simulink model "Joint_Control_r2007a"  (Simulink 6.0)
settings: Solver=ode1  StartTime=0.0  StopTime=inf  FixedStep=0.001  RelTol=1e-3
undefined symbols (not defined in the file): HIL, qc_get_step_size
libraries: simulink x6, quarc_library x3
settings Model: Creator=RSamra  LastModifiedBy=ajavid  SimulationMode=external  ExtModeTrigDuration=10000
settings SolverCC: PositivePriorityOrder=on
settings OptimizationCC: InlineInvariantSignals=off  ExpressionDepthLimit=2147483647  SimCompilerOptimization=Off
settings DebuggingCC: SignalResolutionControl=UseLocalSettings  FcnCallInpInsideContextMsg=Use local settings  StateNameClashWarn=warning  StrictBusMsg=Warning
settings HardwareCC: TargetHWDeviceType=32-bit Generic
settings RTWCC: SystemTargetFile=quarc_windows.tlc  TemplateMakefile=quarc_default_tmf  Description=QuaRC Win32 Target  ProcessScript=quarc_windows_make_rtw_hook  RTWCompilerOptimization=Off
settings CodeAppCC: CustomSymbolStrType=$N$R$M
settings STFCustomTargetCC: TargetFcnLib=ansi_tfl_tmw.mat  TargetPreCompLibLocation=C:\DOCUME~1\ALLUSE~1\APPLIC~1\QuaRC\lib\2007b\windows\release  GenFloatMathFcnCalls=ANSI_C  SystemTargetFile=quarc_windows.tlc
settings GRTTargetCC: TargetPreCompLibLocation=C:\DOCUME~1\ALLUSE~1\APPLIC~1\QuaRC\lib\2007b\windows\release  CompOptLevelCompliant=off  MatFileLogging=off  ExtMode=on  ExtModeMexFile=quarc_comm

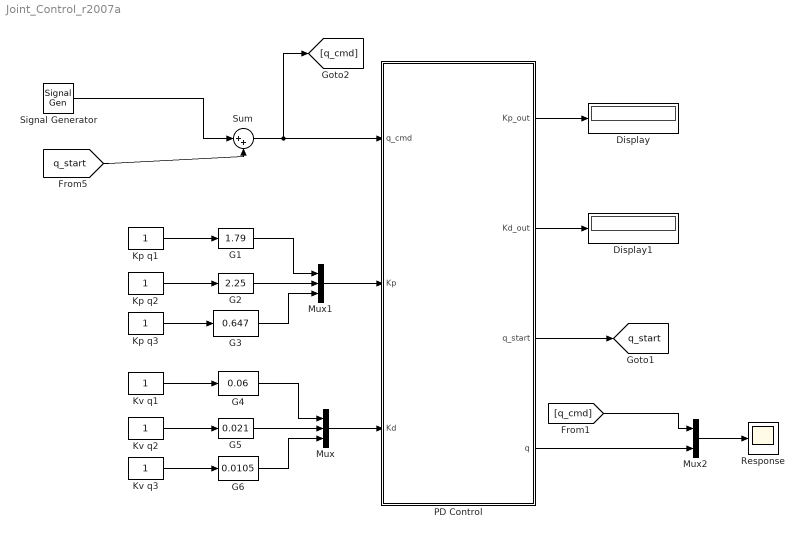
== system Joint_Control_r2007a ==
  Display : Display
  Display1 : Display
  G1 : simulink/Math Operations/Slider Gain  SystemSampleTime=-1  low=0  gain=1.79  high=2
  G2 : simulink/Math Operations/Slider Gain  SystemSampleTime=-1  low=0  gain=2.25  high=3
  G3 : simulink/Math Operations/Slider Gain  SystemSampleTime=-1  low=0  gain=0.647  high=1
  G4 : simulink/Math Operations/Slider Gain  SystemSampleTime=-1  low=0.02  gain=0.06  high=0.1
  G5 : simulink/Math Operations/Slider Gain  SystemSampleTime=-1  low=0.02  gain=0.021  high=0.1
  G6 : simulink/Math Operations/Slider Gain  SystemSampleTime=-1  low=0  gain=0.0105  high=0.025
  Kp q1 : Constant  OutDataType=sfix(16)  OutScaling=2^0
  Kp q2 : Constant  OutDataType=sfix(16)  OutScaling=2^0
  Kp q3 : Constant  OutDataType=sfix(16)  OutScaling=2^0
  Kv q1 : Constant  OutDataType=sfix(16)  OutScaling=2^0
  Kv q2 : Constant  OutDataType=sfix(16)  OutScaling=2^0
  Kv q3 : Constant  OutDataType=sfix(16)  OutScaling=2^0
  Mux : Mux  Inputs=3
  Mux1 : Mux  Inputs=3
  Mux2 : Mux  Inputs=2
  PD Control : Subsystem
  Response : Scope
      settings: TimeRange=50  YMin=-1.25  YMax=3.75
  Signal Generator : SignalGenerator  WaveForm=square  Amplitude=[pi/18 0 0]  Frequency=0.5
  Sum : Sum  Inputs=|++  OutDataType=sfix(16)  OutScaling=2^0
  tag scope: q_start=global
  wires:
  PD Control/3(q_start) -> [q_start]
  Mux2/1 -> Response/1
  Sum/1 -> [q_cmd], PD Control/1(q_cmd)
  [q_start] -> Sum/2
  Signal Generator/1 -> Sum/1
  [q_cmd] -> Mux2/1
  PD Control/4(q) -> Mux2/2
  PD Control/1(Kp_out) -> Display/1
  PD Control/2(Kd_out) -> Display1/1
  Mux/1 -> PD Control/3(Kd)
  Mux1/1 -> PD Control/2(Kp)
  Kp q1/1 -> G1/1
  Kp q2/1 -> G2/1
  Kp q3/1 -> G3/1
  Kv q1/1 -> G4/1
  Kv q2/1 -> G5/1
  Kv q3/1 -> G6/1
  G1/1 -> Mux1/1
  G2/1 -> Mux1/2
  G3/1 -> Mux1/3
  G4/1 -> Mux/1
  G5/1 -> Mux/2
  G6/1 -> Mux/3

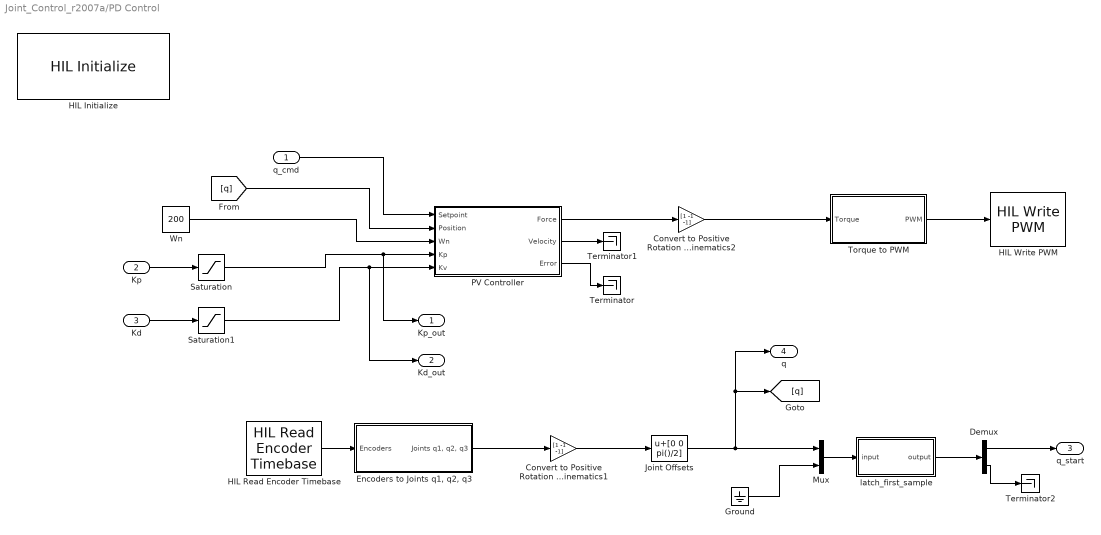
== system Joint_Control_r2007a/PD Control ==
  q_cmd : Inport  OutDataType=sfix(16)  OutScaling=2^0
  Kp : Inport  Port=2  OutDataType=sfix(16)  OutScaling=2^0
  Kd : Inport  Port=3  OutDataType=sfix(16)  OutScaling=2^0
  Convert to Positive Rotation Convension Used in Kinematics1 : Gain  Gain=[1 -1 -1]  ParameterDataType=sfix(16)  ParameterScaling=2^0  OutDataType=sfix(16)  OutScaling=2^0
  Convert to Positive Rotation Convension Used in Kinematics2 : Gain  Gain=[1 -1 -1]  ParameterDataType=sfix(16)  ParameterScaling=2^0  OutDataType=sfix(16)  OutScaling=2^0
  Demux : Demux  Outputs=2
  "Encoders to Joints q1, q2, q3" : Subsystem
  Ground : Ground
  HIL Initialize : quarc_library/Data Acquisition/Generic/Configuration/HIL Initialize  object_name=HIL-3  board_type=phantom_omni  board_number=0  active=on  hardware_clocks=[]  clock_modes=[]  set_clock_params_at_start=off  set_clock_params_at_switch_in=off  analog_input_channels=0:1  analog_input_maximums=10  analog_input_minimums=-10  set_analog_input_params_at_start=off  set_analog_input_params_at_switch_in=off  analog_output_channels=[]  analog_output_maximums=[]  analog_output_minimums=[]  initial_analog_outputs=[]  final_analog_outputs=[]  watchdog_analog_outputs=0  set_analog_output_params_at_start=off  set_analog_output_params_at_switch_in=off  set_analog_outputs_at_start=off  set_analog_outputs_at_switch_in=off  set_analog_outputs_at_terminate=off  set_analog_outputs_at_switch_out=off  set_analog_outputs_on_watchdog=off  digital_input_channels=[]  digital_output_channels=[]  initial_digital_outputs=[]  final_digital_outputs=[]  watchdog_digital_outputs=0  set_digital_outputs_at_start=off  set_digital_outputs_at_switch_in=off  set_digital_outputs_at_terminate=off  set_digital_outputs_at_switch_out=off  set_digital_outputs_on_watchdog=off  encoder_channels=0:2  quadrature=[]  encoder_filter_frequency=[]  initial_encoder_counts=0  set_encoder_params_at_start=off  set_encoder_params_at_switch_in=off  set_encoder_counts_at_start=off  set_encoder_counts_at_switch_in=off  pwm_channels=0:2  pwm_modes=[]  pwm_frequency=[]  initial_pwm_outputs=0  final_pwm_outputs=0  watchdog_pwm_outputs=0  set_pwm_params_at_start=off  set_pwm_params_at_switch_in=off  set_pwm_outputs_at_start=on  set_pwm_outputs_at_switch_in=off  set_pwm_outputs_at_terminate=on  set_pwm_outputs_at_switch_out=off  set_pwm_outputs_on_watchdog=off  other_output_channels=[]  initial_other_outputs=[]  final_other_outputs=[]  watchdog_other_outputs=0  set_other_outputs_at_start=off  set_other_outputs_at_switch_in=off  set_other_outputs_at_terminate=off  set_other_outputs_at_switch_out=off  set_other_outputs_on_watchdog=off
  HIL Read Encoder Timebase : quarc_library/Data Acquisition/Generic/Timebases/HIL Read Encoder Timebase  object_name=HIL-3  clock=0  channels=0:2  samples_in_buffer=max(ceil(1/qc_get_step_size), 1)  active=on  vector_output=on  data_type_mode=Inherit via back propagation  data_type=double
  HIL Write PWM : quarc_library/Data Acquisition/Generic/Immediate I//O/HIL Write PWM  object_name=HIL-3  channels=0:2  sample_time=-1  active=off  vector_input=on
      settings: AttributesFormatString=(%<object_name>)
  Joint Offsets : Bias  Bias=[0 0 pi()/2]
  Mux : Mux  Inputs=2
  PV Controller : Subsystem
  Saturation : Saturate  UpperLimit=[2 2 1]  LowerLimit=[0 0 0]
  Saturation1 : Saturate  UpperLimit=[.1 .1 .025]  LowerLimit=[.02 .02 0]
  Terminator : Terminator
  Terminator1 : Terminator
  Terminator2 : Terminator
  Torque to PWM : Subsystem
  Wn : Constant  Value=200  OutDataType=sfix(16)  OutScaling=2^0
  latch_first_sample : Subsystem
  Kp_out : Outport  OutDataType=sfix(16)  OutScaling=2^0
  Kd_out : Outport  Port=2  OutDataType=sfix(16)  OutScaling=2^0
  q_start : Outport  Port=3  OutDataType=sfix(16)  OutScaling=2^0
  q : Outport  Port=4  OutDataType=sfix(16)  OutScaling=2^0
  wires:
  [q] -> PV Controller/2(Position)
  Wn/1 -> PV Controller/3(Wn)
  Demux/1 -> q_start/1
  Mux/1 -> latch_first_sample/1(input)
  latch_first_sample/1(output) -> Demux/1
  PV Controller/1(Force) -> Convert to Positive Rotation Convension Used in Kinematics2/1
  PV Controller/3(Error) -> Terminator/1
  PV Controller/2(Velocity) -> Terminator1/1
  Ground/1 -> Mux/2
  Demux/2 -> Terminator2/1
  q_cmd/1 -> PV Controller/1(Setpoint)
  Convert to Positive Rotation Convension Used in Kinematics2/1 -> Torque to PWM/1(Torque)
  Convert to Positive Rotation Convension Used in Kinematics1/1 -> Joint Offsets/1
  Joint Offsets/1 -> Mux/1, [q], q/1
  Torque to PWM/1(PWM) -> HIL Write PWM/1
  HIL Read Encoder Timebase/1 -> "Encoders to Joints q1, q2, q3"/1(Encoders)
  "Encoders to Joints q1, q2, q3"/1("Joints q1, q2, q3") -> Convert to Positive Rotation Convension Used in Kinematics1/1
  Kp/1 -> Saturation/1
  Saturation/1 -> PV Controller/4(Kp), Kp_out/1
  Kd/1 -> Saturation1/1
  Saturation1/1 -> PV Controller/5(Kv), Kd_out/1

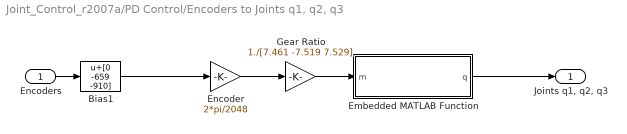
== system Joint_Control_r2007a/PD Control/Encoders to Joints q1, q2, q3 ==
  Encoders : Inport
  Bias1 : Bias  Bias=[0 -659 -910]
  Embedded MATLAB Function : Stateflow chart
      settings: PermitHierarchicalResolution=ParametersOnly
  Encoder : Gain  Gain=2*pi/2048  ParameterDataType=sfix(16)  ParameterScaling=2^0  OutDataType=sfix(16)  OutScaling=2^0
  Gear Ratio : Gain  Gain=1./[7.461 -7.519 7.529]  ParameterDataType=sfix(16)  ParameterScaling=2^0  OutDataType=sfix(16)  OutScaling=2^0
  "Joints q1, q2, q3" : Outport
  wires:
  Embedded MATLAB Function/1(q) -> "Joints q1, q2, q3"/1
  Encoders/1 -> Bias1/1
  Encoder/1 -> Gear Ratio/1
  Gear Ratio/1 -> Embedded MATLAB Function/1(m)
  Bias1/1 -> Encoder/1

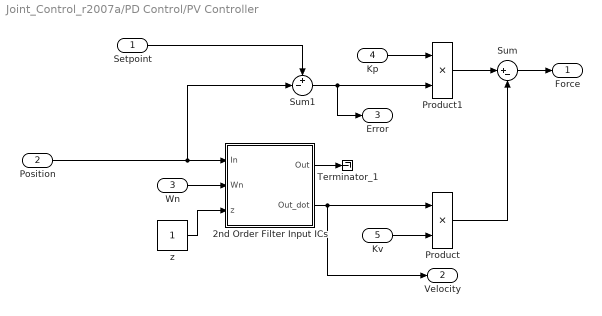
== system Joint_Control_r2007a/PD Control/PV Controller ==
  Setpoint : Inport  OutDataType=sfix(16)  OutScaling=2^0
  Position : Inport  Port=2  OutDataType=sfix(16)  OutScaling=2^0
  Wn : Inport  Port=3  OutDataType=sfix(16)  OutScaling=2^0
  Kp : Inport  Port=4  OutDataType=sfix(16)  OutScaling=2^0
  Kv : Inport  Port=5  OutDataType=sfix(16)  OutScaling=2^0
  2nd Order Filter Input ICs : Subsystem
  Product : Product  OutDataType=sfix(16)  OutScaling=2^0  RndMeth=Zero
  Product1 : Product  OutDataType=sfix(16)  OutScaling=2^0  RndMeth=Zero
  Sum : Sum  Inputs=|+-  OutDataType=sfix(16)  OutScaling=2^0
  Sum1 : Sum  Inputs=+-|  OutDataType=sfix(16)  OutScaling=2^0
  Terminator_1 : Terminator
  z : Constant  OutDataType=sfix(16)  OutScaling=2^0
  Force : Outport  OutDataType=sfix(16)  OutScaling=2^0
  Velocity : Outport  Port=2  OutDataType=sfix(16)  OutScaling=2^0
  Error : Outport  Port=3  OutDataType=sfix(16)  OutScaling=2^0
  wires:
  Wn/1 -> 2nd Order Filter Input ICs/2(Wn)
  z/1 -> 2nd Order Filter Input ICs/3(z)
  Position/1 -> 2nd Order Filter Input ICs/1(In), Sum1/2
  2nd Order Filter Input ICs/2(Out_dot) -> Velocity/1, Product/1
  Kp/1 -> Product1/1
  Setpoint/1 -> Sum1/1
  Sum1/1 -> Product1/2, Error/1
  Product1/1 -> Sum/1
  Kv/1 -> Product/2
  Product/1 -> Sum/2
  Sum/1 -> Force/1
  2nd Order Filter Input ICs/1(Out) -> Terminator_1/1

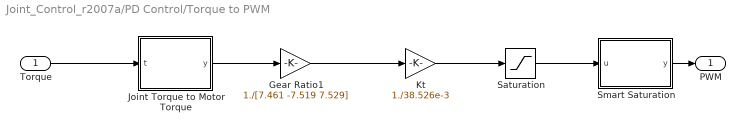
== system Joint_Control_r2007a/PD Control/Torque to PWM ==
  Torque : Inport
  Gear Ratio1 : Gain  Gain=1./[7.461 -7.519 7.529]  ParameterDataType=sfix(16)  ParameterScaling=2^0  OutDataType=sfix(16)  OutScaling=2^0
  Joint Torque to Motor Torque : Stateflow chart
      settings: PermitHierarchicalResolution=ParametersOnly
  Kt : Gain  Gain=1./38.526e-3  ParameterDataType=sfix(16)  ParameterScaling=2^0  OutDataType=sfix(16)  OutScaling=2^0
  Saturation : Saturate  UpperLimit=1.6  LowerLimit=-1.6
  Smart Saturation : Stateflow chart
      settings: PermitHierarchicalResolution=ParametersOnly
  PWM : Outport
  wires:
  Torque/1 -> Joint Torque to Motor Torque/1(t)
  Smart Saturation/1(y) -> PWM/1
  Saturation/1 -> Smart Saturation/1(u)
  Kt/1 -> Saturation/1
  Gear Ratio1/1 -> Kt/1
  Joint Torque to Motor Torque/1(y) -> Gear Ratio1/1

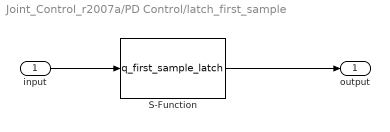
== system Joint_Control_r2007a/PD Control/latch_first_sample ==
  input : Inport  OutDataType=sfix(16)  OutScaling=2^0
  S-Function : S-Function  FunctionName=q_first_sample_latch  SFunctionModules=q_first_sample_latch_wrapper
  output : Outport  OutDataType=sfix(16)  OutScaling=2^0
  wires:
  input/1 -> S-Function/1
  S-Function/1 -> output/1

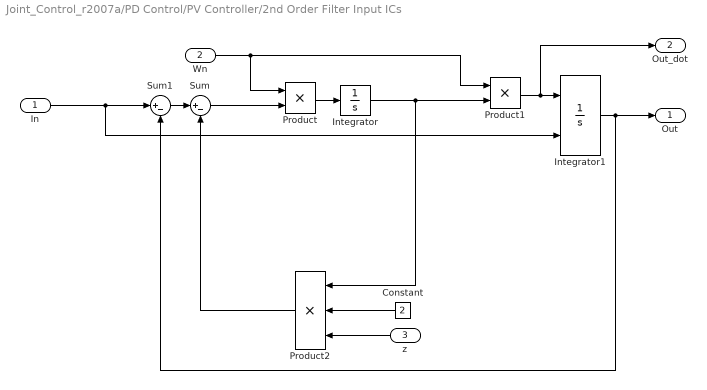
== system Joint_Control_r2007a/PD Control/PV Controller/2nd Order Filter Input ICs ==
  In : Inport  OutDataType=sfix(16)  OutScaling=2^0
  Wn : Inport  Port=2  OutDataType=sfix(16)  OutScaling=2^0
  z : Inport  Orientation=left  Port=3  OutDataType=sfix(16)  OutScaling=2^0
  Constant : Constant  Orientation=left  Value=2  OutDataType=sfix(16)  OutScaling=2^0
  Integrator : Integrator
  Integrator1 : Integrator  InitialConditionSource=external
  Product : Product  OutDataType=sfix(16)  OutScaling=2^0  RndMeth=Zero
  Product1 : Product  OutDataType=sfix(16)  OutScaling=2^0  RndMeth=Zero
  Product2 : Product  Orientation=left  Inputs=3  OutDataType=sfix(16)  OutScaling=2^0  RndMeth=Zero
  Sum : Sum  Inputs=|+-  OutDataType=sfix(16)  OutScaling=2^0
  Sum1 : Sum  Inputs=|+-  OutDataType=sfix(16)  OutScaling=2^0
  Out : Outport  OutDataType=sfix(16)  OutScaling=2^0
  Out_dot : Outport  Port=2  OutDataType=sfix(16)  OutScaling=2^0
  wires:
  Constant/1 -> Product2/2
  z/1 -> Product2/3
  Product2/1 -> Sum/2
  In/1 -> Integrator1/2, Sum1/1
  Sum1/1 -> Sum/1
  Integrator1/1 -> Out/1, Sum1/2
  Integrator/1 -> Product2/1, Product1/2
  Product1/1 -> Out_dot/1, Integrator1/1
  Wn/1 -> Product1/1, Product/1
  Sum/1 -> Product/2
  Product/1 -> Integrator/1

== matlab function PD Control/Torque to PWM/Smart Saturation ==
  data: u input inherited; y output inherited size=3
function y = fcn(u)
% Smart Saturation: allows channels to go up to 1.6A 
% unless the total exceeds 2.2A in which case all channels
% are scaled so that the cumulative current is equal to 2.2A.

y = zeros(3,1);
MAX_CURRENT = 2.2; % Define the maximum cumulative current here

total = sum(abs(u));
if (total > MAX_CURRENT)
    y = MAX_CURRENT/total*u;
else
    y = u;
end

== matlab function PD Control/Torque to PWM/Joint Torque to Motor Torque ==
  data: t input inherited; y output inherited
function y = fcn( t)
% Smart Saturation: allows channels to go up to 1.6A 
% unless the total exceeds 2.2A in which case all channels
% are scaled so that the cumulative current is equal to 2.2A.
y=[0 0 0]'

y(1)=t(1);
y(3)=t(3);
y(2)=t(2)-t(3);


end

== matlab function PD Control/Encoders to Joints q1, q2, q3/Embedded MATLAB Function ==
  data: m input inherited; q output inherited
function q = Motors_2_Joints(m)
q = m;
q(1) = m(1);
q(2) = m(2);
q(3) = m(3) - m(2) -pi/2;
end
